simulink model "FMI3"  (R2023b)
settings: Solver=VariableStepAuto  StartTime=0.0  StopTime=inf  RelTol=1e-3
undefined symbols (not defined in the file): BeamNG, FMI3
settings Model: Creator=User  LastModifiedBy=User
settings OptimizationCC: ReuseModelBlockBuffer=off

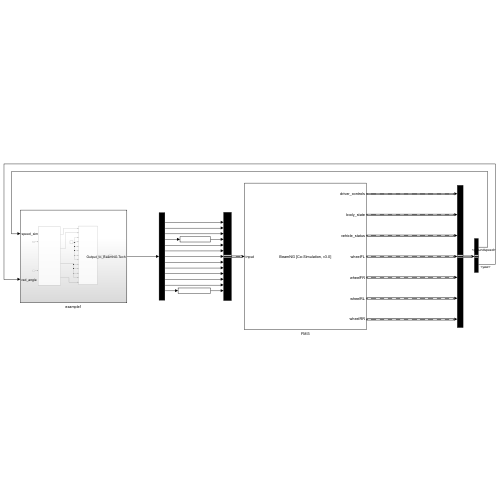
[thumbnail: Simulink's stored preview of the top-level diagram]
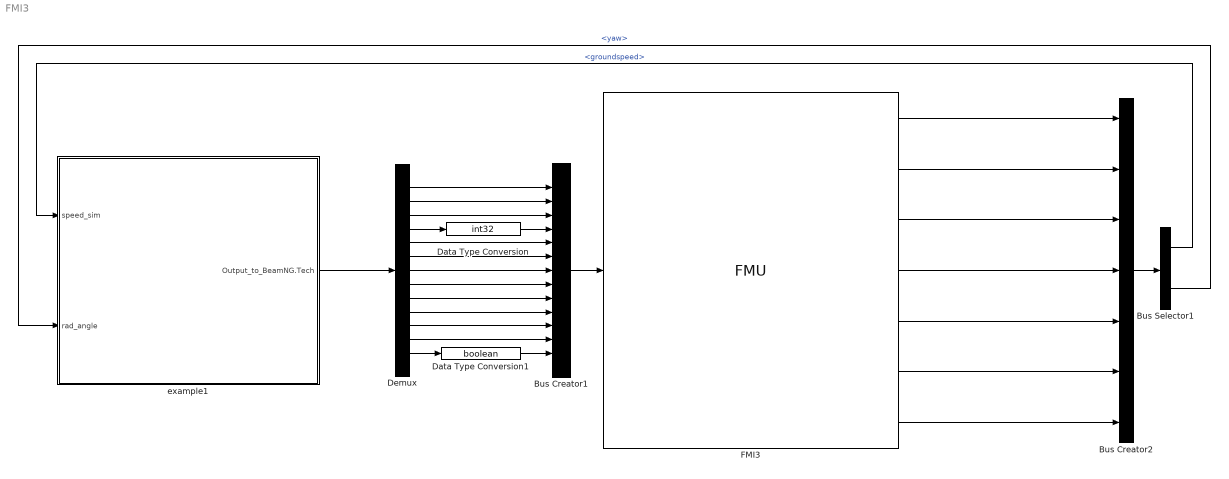
== system FMI3 ==
  Bus Creator1 : BusCreator  Inputs=13  OutDataTypeStr=Bus: input  NonVirtualBus=on
  Bus Creator2 : BusCreator  Inputs=7
  Bus Selector1 : BusSelector  OutputSignals=signal2.groundspeed,signal2.yaw
  Data Type Conversion : DataTypeConversion  OutDataTypeStr=int32  SaturateOnIntegerOverflow=off  RndMeth=Floor
  Data Type Conversion1 : DataTypeConversion  OutDataTypeStr=boolean  SaturateOnIntegerOverflow=off  RndMeth=Floor
  Demux : Demux  Outputs=13
  FMI3 : FMU  FMUName=BeamNG-FMI3.fmu  FMUMode=CoSimulation  FMUCachedDialogLayout="{\"Geometry\":[37,234,544,434],\"ParameterColumnsWidthConfig\":\"{\\\"columns\\\":[{\\\"name\\\":\\\"Parameter\\\",\\\"width\\\":219},{\\\"name\\\":\\\"Value\\\",\\\"width\\\":178},{\\\"name\\\":\\\"Unit\\\",\\\"width\\\":168},{\\\"name\\\":\\\"Description\\\",\\\"width\\\":231}]}\",\"InputColumnsWidthConfig\":[],\"OutputColumnsWidthConfig\":[]}"  socket=struct('inPort',int32(64890),'outPort',int32(64891))  socket_inAddress=127.0.0.1  socket_outAddress=127.0.0.1  mask(BeamNG [Co-Simulation, v3.0]){}
      mask Display:
      | disp('BeamNG [Co-Simulation, v3.0]');
      | port_label('output',1,'driver_controls');
      | port_label('output',2,'body_state');
      | port_label('output',3,'vehicle_status');
      | port_label('output',4,'wheelFL');
      | port_label('output',5,'wheelFR');
      | port_label('output',6,'wheelRL');
      | port_label('output',7,'wheelRR');
      | port_label('input',1,'input');
  example1 : Subsystem
  wires:
  Bus Creator1/1 -> FMI3/1
  Bus Creator2/1 -> Bus Selector1/1
  Demux/13 -> Data Type Conversion1/1
  Demux/8 -> Bus Creator1/8
  Demux/6 -> Bus Creator1/6
  Demux/9 -> Bus Creator1/9
  Data Type Conversion1/1 -> Bus Creator1/13
  Demux/4 -> Data Type Conversion/1
  Demux/3 -> Bus Creator1/3
  Demux/10 -> Bus Creator1/10
  Demux/7 -> Bus Creator1/7
  Data Type Conversion/1 -> Bus Creator1/4
  Demux/11 -> Bus Creator1/11
  Demux/12 -> Bus Creator1/12
  Bus Selector1/2 -> example1/2(rad_angle)  "<yaw>"
  Demux/5 -> Bus Creator1/5
  example1/1(Output_to_BeamNG.Tech) -> Demux/1
  Bus Selector1/1 -> example1/1(speed_sim)  "<groundspeed>"
  FMI3/1 -> Bus Creator2/1
  Demux/1 -> Bus Creator1/1
  FMI3/5 -> Bus Creator2/5
  FMI3/4 -> Bus Creator2/4
  FMI3/2 -> Bus Creator2/2
  FMI3/3 -> Bus Creator2/3
  Demux/2 -> Bus Creator1/2
  FMI3/6 -> Bus Creator2/6
  FMI3/7 -> Bus Creator2/7

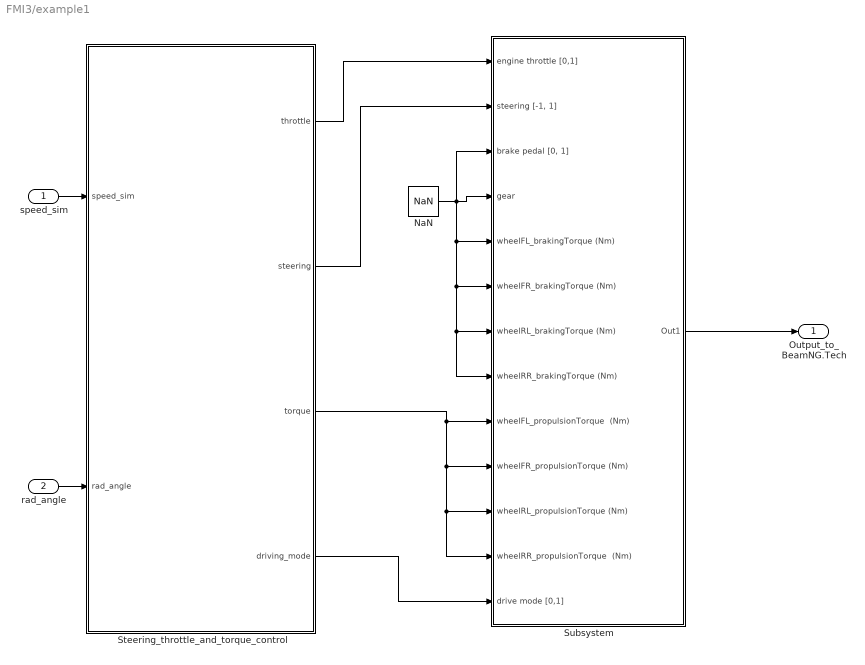
== system FMI3/example1 ==
  speed_sim : Inport
  rad_angle : Inport  Port=2
  NaN : Constant  Value=NaN  OutDataTypeStr=Inherit: Inherit via back propagation
  Steering_throttle_and_torque_control : Subsystem
  Subsystem : Subsystem
  Output_to_BeamNG.Tech : Outport
  wires:
  rad_angle/1 -> Steering_throttle_and_torque_control/2(rad_angle)
  Subsystem/1(Out1) -> Output_to_BeamNG.Tech/1
  speed_sim/1 -> Steering_throttle_and_torque_control/1(speed_sim)
  Steering_throttle_and_torque_control/3(torque) -> Subsystem/10(wheelFR_propulsionTorque (Nm)), Subsystem/11(wheelRL_propulsionTorque (Nm)), Subsystem/12(wheelRR_propulsionTorque	 (Nm)), Subsystem/9(wheelFL_propulsionTorque	 (Nm))
  Steering_throttle_and_torque_control/4(driving_mode) -> Subsystem/13(drive mode [0,1])
  Steering_throttle_and_torque_control/2(steering) -> Subsystem/2("steering\t[-1, 1]")
  Steering_throttle_and_torque_control/1(throttle) -> Subsystem/1("engine throttle [0,1] ")
  NaN/1 -> Subsystem/3("brake pedal [0, 1]"), Subsystem/8("wheelRR_brakingTorque (Nm)\t"), Subsystem/7("wheelRL_brakingTorque (Nm)\t"), Subsystem/6("wheelFR_brakingTorque (Nm)\t"), Subsystem/5("wheelFL_brakingTorque (Nm)\t"), Subsystem/4("gear ")

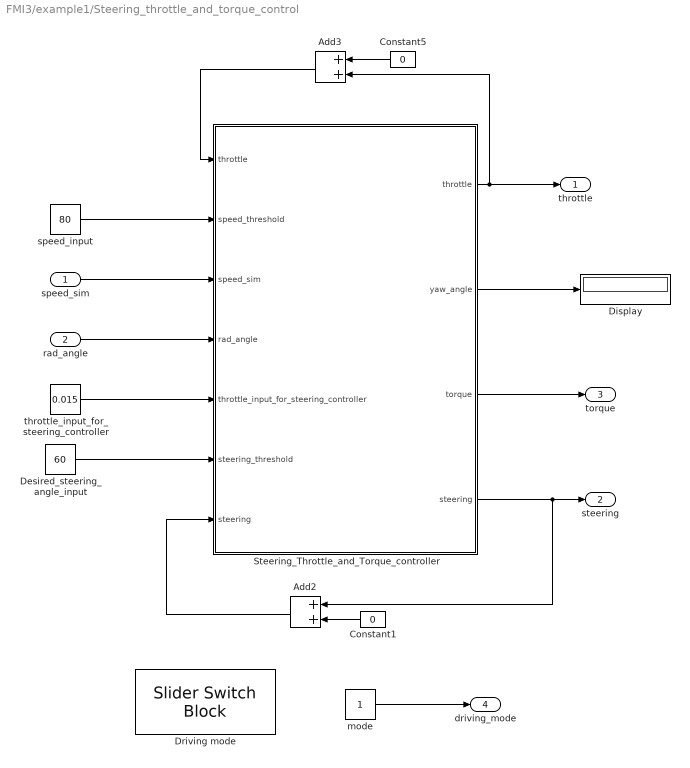
== system FMI3/example1/Steering_throttle_and_torque_control ==
  speed_sim : Inport
  rad_angle : Inport  Port=2
  Add2 : Sum
  Add3 : Sum
  Constant1 : Constant  Value=0
  Constant5 : Constant  Value=0
  Desired_steering_angle_input : Constant  Value=60
  Display : Display
  Driving mode : SliderSwitchBlock
      settings: Values={{'Torque', 'Pedal'}, [1 0]}
  Steering_Throttle_and_Torque_controller : MATLAB Function  TreatAsAtomicUnit=on
  mode : Constant
  speed_input : Constant  Value=80
  throttle_input_for_steering_controller : Constant  Value=0.015
  throttle : Outport
  steering : Outport  Port=2
  torque : Outport  Port=3
  driving_mode : Outport  Port=4  OutDataTypeStr=double
  wires:
  speed_input/1 -> Steering_Throttle_and_Torque_controller/2(speed_threshold)
  Desired_steering_angle_input/1 -> Steering_Throttle_and_Torque_controller/6(steering_threshold)
  Constant5/1 -> Add3/1
  Steering_Throttle_and_Torque_controller/1(throttle) -> Add3/2, throttle/1
  Add2/1 -> Steering_Throttle_and_Torque_controller/7("steering ")
  Constant1/1 -> Add2/2
  Add3/1 -> Steering_Throttle_and_Torque_controller/1("throttle ")
  mode/1 -> driving_mode/1
  Steering_Throttle_and_Torque_controller/3(torque) -> torque/1
  Steering_Throttle_and_Torque_controller/4(steering) -> Add2/1, steering/1
  rad_angle/1 -> Steering_Throttle_and_Torque_controller/4(rad_angle)
  speed_sim/1 -> Steering_Throttle_and_Torque_controller/3(speed_sim)
  throttle_input_for_steering_controller/1 -> Steering_Throttle_and_Torque_controller/5(throttle_input_for_steering_controller)
  Steering_Throttle_and_Torque_controller/2(yaw_angle) -> Display/1

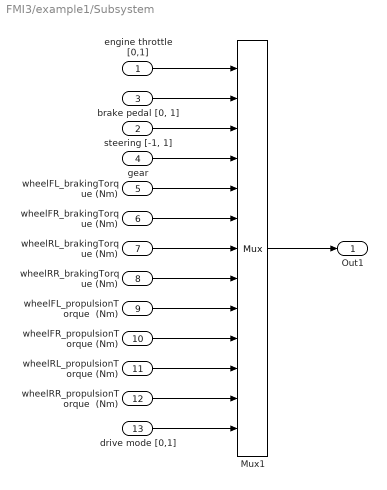
== system FMI3/example1/Subsystem ==
  "engine throttle [0,1] " : Inport
  "steering\t[-1, 1]" : Inport  Port=2
  "brake pedal [0, 1]" : Inport  Port=3
  "gear " : Inport  Port=4
  "wheelFL_brakingTorque (Nm)\t" : Inport  Port=5
  "wheelFR_brakingTorque (Nm)\t" : Inport  Port=6
  "wheelRL_brakingTorque (Nm)\t" : Inport  Port=7
  "wheelRR_brakingTorque (Nm)\t" : Inport  Port=8
  wheelFL_propulsionTorque	 (Nm) : Inport  Port=9
  wheelFR_propulsionTorque (Nm) : Inport  Port=10
  wheelRL_propulsionTorque (Nm) : Inport  Port=11
  wheelRR_propulsionTorque	 (Nm) : Inport  Port=12
  drive mode [0,1] : Inport  Port=13
  Mux1 : Mux  Inputs=13
  Out1 : Outport
  wires:
  "wheelFR_brakingTorque (Nm)\t"/1 -> Mux1/6
  "wheelRL_brakingTorque (Nm)\t"/1 -> Mux1/7
  "wheelRR_brakingTorque (Nm)\t"/1 -> Mux1/8
  "brake pedal [0, 1]"/1 -> Mux1/2
  drive mode [0,1]/1 -> Mux1/13
  wheelRR_propulsionTorque	 (Nm)/1 -> Mux1/12
  wheelFR_propulsionTorque (Nm)/1 -> Mux1/10
  wheelRL_propulsionTorque (Nm)/1 -> Mux1/11
  "wheelFL_brakingTorque (Nm)\t"/1 -> Mux1/5
  "engine throttle [0,1] "/1 -> Mux1/1
  "gear "/1 -> Mux1/4
  "steering\t[-1, 1]"/1 -> Mux1/3
  wheelFL_propulsionTorque	 (Nm)/1 -> Mux1/9
  Mux1/1 -> Out1/1

== matlab function FMI3/example1/Steering_throttle_and_torque_control/Steering_Throttle_and_Torque_controller ==
  data: throttle input; throttle output; yaw_angle output; torque output; steering output; speed_threshold input; speed_sim input; rad_angle input; throttle_input_for_steering_controller input; steering_threshold input; steering input
function [throttle,yaw_angle,torque,steering]= Controller(throttle,speed_threshold,speed_sim,rad_angle,throttle_input_for_steering_controller,steering_threshold,steering)
    % Steering 
    steering_clearance=1; % in degrees
    % here's converting the angle from radiant to degree      
    yaw_angle=rad_angle*(180/pi);
    if yaw_angle <= (steering_threshold-steering_clearance)
    steering=-throttle_input_for_steering_controller;
    end   

    if  yaw_angle > (steering_threshold)
    steering=throttle_input_for_steering_controller;
    end   


    % Throttle and Torque 
    speed_clearance=10;
    actual_speed=speed_sim*3.6;
    if actual_speed <= 5
    torque = 270 ; 
    throttle=0.5;
    elseif actual_speed <= (speed_threshold-speed_clearance)
    throttle=0.5;
    torque = 200 ; 
    elseif  actual_speed > (speed_threshold)
    throttle=-0.05;
    torque = 65; 
    else
    torque = 170; 
    end
    end
